simulink model "IMU_Model"  (R2024a)
settings: Solver=FixedStepDiscrete  StartTime=0.0  StopTime=inf  FixedStep=0.1  RelTol=1e-3  EnableMultiTasking=on
libraries: simulink x2
settings Model: Creator=matat  LastModifiedBy=matat
settings SolverCC: AlgebraicLoopSolver=TrustRegion  AutoInsertRateTranBlk=on
settings DataIOCC: LimitDataPoints=on
settings OptimizationCC: LifeSpan=inf
settings DebuggingCC: UnconnectedInputMsg=warning  UnconnectedOutputMsg=warning  UnconnectedLineMsg=warning  AllowSymbolicDim=off  SFUnexpectedBacktrackingDiag=warning  SFNoUnconditionalDefaultTransitionDiag=warning  SFExecutionAtInitializationDiag=none  ArithmeticOperatorsInVariantConditions=warning
settings ModelReferenceCC: EnableRefExpFcnMdlSchedulingChecks=on
settings SFSimCC: SimUseLocalCustomCode=off  CustomCodeUndefinedFunction=UseInterfaceOnly
settings RTWCC: RTWUseLocalCustomCode=off  GPUComputeCapability=3.5  DLArmComputeVersion=19.05
settings CodeAppCC: StateflowObjectComments=on
settings GRTTargetCC: TargetLangStandard=C89/C90 (ANSI)
settings ConfigComp: CovMetricSettings=dw  CovSaveCumulativeToWorkspaceVar=on  CovSaveSingleToWorkspaceVar=on  CovExternalEMLEnable=off  CovSFcnEnable=off

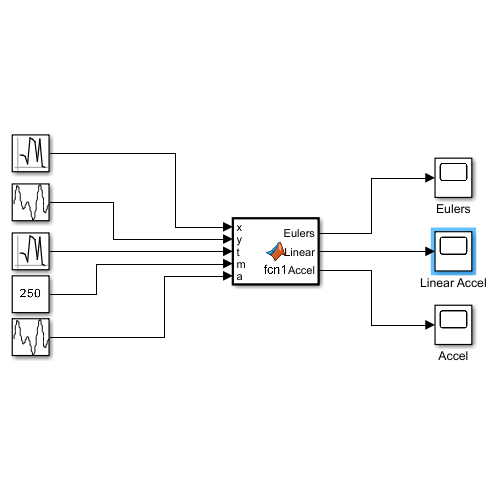
[thumbnail: Simulink's stored preview of the top-level diagram]
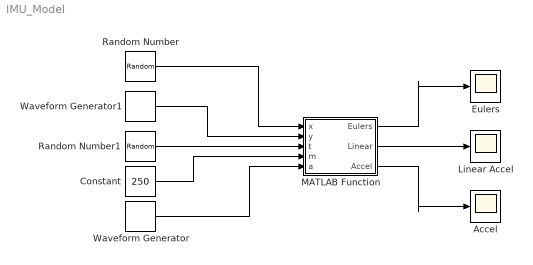
== system IMU_Model ==
  Accel : Scope
  Constant : Constant  Value=250
  Eulers : Scope
  Linear Accel : Scope
  MATLAB Function : MATLAB Function  TreatAsAtomicUnit=on
  Random Number : RandomNumber  Variance=5  SampleTime=0.1
  Random Number1 : RandomNumber  Variance=5  SampleTime=0.1
  Waveform Generator : simulink/Sources/Waveform Generator  OutMin=[]  OutMax=[]  OutDataTypeStr=double  SelectedSignal=1  Signals=abs(sin(1, 3, 1))  BlockNames=MultiportSwitch_f75b000729e840e  SampleTime=0.1
  Waveform Generator1 : simulink/Sources/Waveform Generator  OutMin=[]  OutMax=[]  OutDataTypeStr=double  SelectedSignal=1  Signals=abs(sin(1, 1, 1))  BlockNames=MultiportSwitch_399d56559a454e8  SampleTime=0.1
  wires:
  MATLAB Function/1(Eulers) -> Eulers/1
  Random Number/1 -> MATLAB Function/1(x)
  Waveform Generator1/1 -> MATLAB Function/2(y)
  MATLAB Function/2(Linear) -> Linear Accel/1
  MATLAB Function/3(Accel) -> Accel/1
  Constant/1 -> MATLAB Function/4(m)
  Waveform Generator/1 -> MATLAB Function/5(a)
  Random Number1/1 -> MATLAB Function/3(t)

== matlab function IMU_Model/MATLAB Function ==
  data: x input; Eulers output; Linear output; Accel output; y input; t input; m input; a input
function [Eulers, Linear, Accel] = fcn1(x, y, t, m ,a)
Eulers = cos(x) + 1i*sin(x); %% Eulers formula 
Linear = (y/t); %% Linear Acceleration formula 
Accel = m*a; %% Accelerometer formula
%% each formula takes random variables and showcases the expected outputs for each function on the board
